simulink model "nonlineare_2_sim"  (Simulink 7.6)
settings: Solver=ode45  StartTime=0.0  StopTime=50  RelTol=1e-3
undefined symbols (not defined in the file): x0
libraries: simulink x1
settings Model: Creator=professore  LastModifiedBy=patrizio
settings OptimizationCC: InlineInvariantSignals=on  InitFltsAndDblsToZero=on
settings DebuggingCC: SaveWithParameterizedLinksMsg=none  SignalResolutionControl=TryResolveAllWithWarning  MultiTaskDSMMsg=warning  MultiTaskCondExecSysMsg=none  StrictBusMsg=None
settings RTWCC: IncludeERTFirstTime=on
settings GRTTargetCC: TargetFcnLib=ansi_tfl_tmw.mat

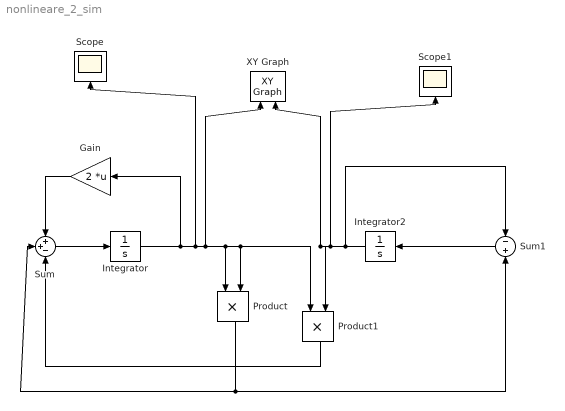
== system nonlineare_2_sim ==
  Gain : Gain  Gain=2  Multiplication=Matrix(K*u)
  Integrator : Integrator  InitialCondition=x0(1)
  Integrator2 : Integrator  InitialCondition=x0(2)
  Product : Product  RndMeth=Zero
  Product1 : Product  RndMeth=Zero
  Scope : Scope
  Scope1 : Scope
  Sum : Sum  Inputs=++-
  Sum1 : Sum  Inputs=-+
  XY Graph : simulink/Sinks/XY Graph  SystemSampleTime=-1  xmin=-10  xmax=10  ymin=-10  ymax=10  st=-1
  wires:
  Integrator/1 -> Gain/1, Product/1, Product/2, Product1/1, XY Graph/1, Scope/1
  Gain/1 -> Sum/1
  Product/1 -> Sum/2, Sum1/2
  Integrator2/1 -> Sum1/1, Product1/2, XY Graph/2, Scope1/1
  Product1/1 -> Sum/3
  Sum/1 -> Integrator/1
  Sum1/1 -> Integrator2/1
